simulink model "MPCmodel"  (R2023b)
settings: Solver=VariableStepAuto  StartTime=0.0  StopTime=10.0  RelTol=1e-3
libraries: aerolibanimutils x1
settings Model: Creator=Lingf  LastModifiedBy=deandre
settings SolverCC: AlgebraicLoopSolver=TrustRegion
settings DebuggingCC: UnconnectedInputMsg=warning  UnconnectedOutputMsg=warning  UnconnectedLineMsg=warning
settings ModelReferenceCC: EnableRefExpFcnMdlSchedulingChecks=on
settings RTWCC: DLArmComputeVersion=19.05

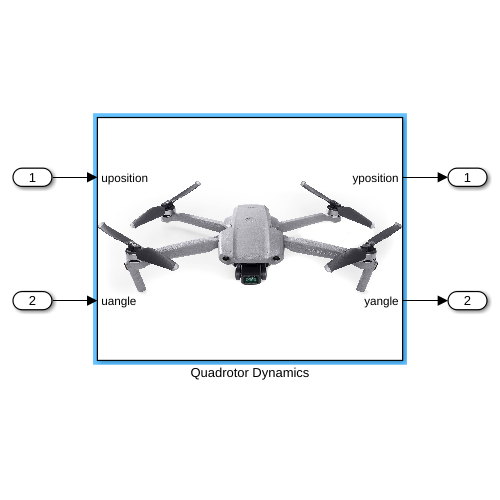
[thumbnail: Simulink's stored preview of the top-level diagram]
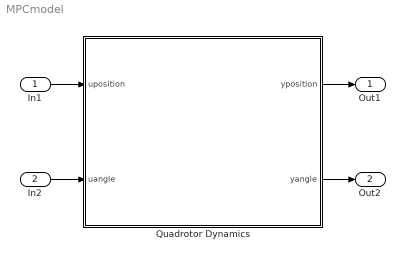
== system MPCmodel ==
  In1 : Inport
  In2 : Inport  Port=2
  Quadrotor Dynamics : Subsystem
      mask Display: image('$imagefile'); % Use "Edit Image" on toolstrip to change.
  Out1 : Outport
  Out2 : Outport  Port=2
  wires:
  In1/1 -> Quadrotor Dynamics/1(uposition)
  In2/1 -> Quadrotor Dynamics/2(uangle)
  Quadrotor Dynamics/1(yposition) -> Out1/1
  Quadrotor Dynamics/2(yangle) -> Out2/1

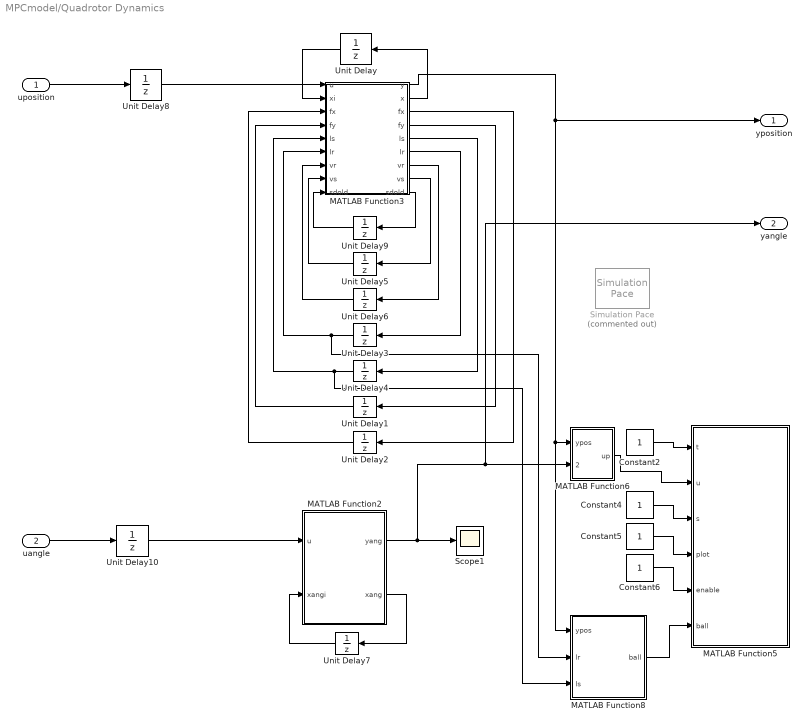
== system MPCmodel/Quadrotor Dynamics ==
  uposition : Inport
  uangle : Inport  Port=2
  Constant{2,4..6} (4 alike) : Constant
  MATLAB Function2 : MATLAB Function  TreatAsAtomicUnit=on
  MATLAB Function3 : MATLAB Function  TreatAsAtomicUnit=on
  MATLAB Function5 : MATLAB Function  TreatAsAtomicUnit=on
  MATLAB Function6 : MATLAB Function  TreatAsAtomicUnit=on
  MATLAB Function8 : MATLAB Function  TreatAsAtomicUnit=on
  Scope1 : Scope
  Simulation Pace : aerolibanimutils/Simulation Pace  Commented=on  SimulationPace=1  SleepMode=Auto  OutputPaceError=off  SampleTime=-1
  Unit Delay : UnitDelay  InitialCondition=|  SampleTime=-1  HasFrameUpgradeWarning=on
      | [0
      | 0
      | 0
      | 0
      | 1.50000000000000
      | 0]
  Unit Delay{1..6,9} (7 alike) : UnitDelay  SampleTime=-1  HasFrameUpgradeWarning=on
  Unit Delay10 : UnitDelay  InitialCondition=|  SampleTime=-1  HasFrameUpgradeWarning=on
      | [0
      | 0
      | 0]
  Unit Delay7 : UnitDelay  InitialCondition=|  SampleTime=-1  HasFrameUpgradeWarning=on
      | [0
      | 0
      | 0
      | 0
      | 0
      | 0]
  Unit Delay8 : UnitDelay  InitialCondition=|  SampleTime=-1  HasFrameUpgradeWarning=on
      | [0
      | 0
      | 0]
  yposition : Outport
  yangle : Outport  Port=2
  wires:
  Unit Delay6/1 -> MATLAB Function3/7("vr ")
  MATLAB Function3/2(x) -> Unit Delay/1
  MATLAB Function3/5(ls) -> Unit Delay4/1
  MATLAB Function2/1(yang) -> Scope1/1, yangle/1, MATLAB Function6/2(yang)
  Constant4/1 -> MATLAB Function5/3(s)
  Constant2/1 -> MATLAB Function5/1(t)
  MATLAB Function3/4(fy) -> Unit Delay1/1
  Unit Delay/1 -> MATLAB Function3/2(xi)
  MATLAB Function3/9(sdold) -> Unit Delay9/1
  MATLAB Function8/1(ball) -> MATLAB Function5/6(ball)
  Unit Delay4/1 -> MATLAB Function8/3(ls), MATLAB Function3/5("ls ")
  Unit Delay2/1 -> MATLAB Function3/3("fx ")
  MATLAB Function2/2(xang) -> Unit Delay7/1
  MATLAB Function3/1(y) -> yposition/1, MATLAB Function8/1(ypos), MATLAB Function6/1(ypos)
  MATLAB Function3/6(lr) -> Unit Delay3/1
  Constant5/1 -> MATLAB Function5/4(plot)
  MATLAB Function3/8(vs) -> Unit Delay5/1
  Unit Delay3/1 -> MATLAB Function8/2(lr), MATLAB Function3/6("lr ")
  Unit Delay5/1 -> MATLAB Function3/8("vs ")
  Constant6/1 -> MATLAB Function5/5(enable)
  MATLAB Function6/1(up) -> MATLAB Function5/2(u)
  Unit Delay7/1 -> MATLAB Function2/2(xangi)
  MATLAB Function3/7(vr) -> Unit Delay6/1
  MATLAB Function3/3(fx) -> Unit Delay2/1
  Unit Delay9/1 -> MATLAB Function3/9("sdold ")
  Unit Delay1/1 -> MATLAB Function3/4("fy ")
  uposition/1 -> Unit Delay8/1
  uangle/1 -> Unit Delay10/1
  Unit Delay8/1 -> MATLAB Function3/1(u)
  Unit Delay10/1 -> MATLAB Function2/1(u)

== matlab function MPCmodel/Quadrotor Dynamics/MATLAB Function2 ==
  data: yang output; xang output; u input; xangi input
function [yang,xang]= sysang(u,xangi)
Ts = 1/40;
g = 9.81;
A = [1,0.0250000000000000,0,0,0,0;0,1,0,0,0,0;0,0,1,0.0250000000000000,0,0;0,0,0,1,0,0;0,0,0,0,1,0.0250000000000000;0,0,0,0,0,1];
B = [0.0416666666666667,0,0;3.33333333333333,0,0;0,0.0416666666666667,0;0,3.33333333333333,0;0,0,0.0240384615384615;0,0,1.92307692307692];
C = [1,0,0,0,0,0;0,0,1,0,0,0;0,0,0,0,1,0];
D = zeros(3,3);
xang = zeros(6,1);
yang = zeros(3,1);
xang = A*xangi + B*u;
yang = C*xang + D*u;

== matlab function MPCmodel/Quadrotor Dynamics/MATLAB Function3 ==
  data: y output; x output; u input; xi input; fx input; fy input; fx output; fy output; ls input; lr input; ls output; lr output; vr input; vs input; vr output; vs output; sdold input; sdold output
function [y,x, fx,fy,ls,lr,vr,vs,sdold]= syspos(u,xi,fx,fy,ls,lr,vr,vs,sdold)
Ts = 1/40;
g = 9.81;
A = [1 0.025 0 0 0 0;0 1 0 0 0 0;0 0 1 0.025 0 0;0 0 0 1 0 0;0 0 0 0 1 0.025;0 0 0 0 0 1];
B = [-0.003065625 0 0;-0.24525 0 0;0 0.003065625 0;0 0.24525 0;0 0 0.0003125;0 0 0.025];
C = [1 0 0 0 0 0;0 0 1 0 0 0;0 0 0 0 1 0];
D = zeros(3,3);
x = zeros(6,1);
y = zeros(3,1);
x = A*xi + B*u;
y = C*x + D*u;
x(2) = x(2) - fx;
x(4) = x(4) - fy;


xdold = x(2)-xi(2);
ydold = x(4)-xi(4);
zdold = x(6)-xi(6);

yita = sqrt(0.5^2-lr^2-ls^2);
vrold = vr;
vsold = vs;
vr = ( yita^4*xdold - lr*yita^3*zdold + lr*ls*yita^2*sdold +...
    (lr*0.5^2-lr*ls^2)*vr^2 +...
    (lr*0.5^2-lr^3)*vs^2 +...
    2*vr*vs*lr^2*ls + lr*g*yita^3 )/((ls^2-0.5^2)*yita^2);
lr = lr + vr*Ts;
rdold = vr-vrold;

vs = ( yita^4*ydold - ls*yita^3*zdold + lr*ls*yita^2*rdold +...
    (ls*0.5^2-ls*lr^2)*vs^2 +...
    (ls*0.5^2-ls^3)*vr^2 +...
    2*vr*vs*ls^2*lr + ls*g*yita^3 )/((lr^2-0.5^2)*yita^2);
ls = ls + vs*Ts;
% sdold = vs(1,i+1);
sdold = vs(1)-vsold(1);

fx = 0.3*(xdold+rdold);
fy = 0.3*(ydold+sdold);

== matlab function MPCmodel/Quadrotor Dynamics/MATLAB Function5 ==
  data: t input; u input; s input; plot input; enable input; ball input
function qd_plot(t,u,s, plot, enable,ball)
    quad.nrotors =4;
    quad.d = 0.17;
    quad.r = 0.1;
    
    a1s = zeros(1, quad.nrotors);
    b1s = zeros(1, quad.nrotors);

    
    % vehicle dimensons
    d = quad.d; %Hub displacement from COG
    r = quad.r; %Rotor radius
    D = zeros(3,4);
    C = zeros(3,4);
    for i = 1:quad.nrotors
        theta = (i-1)/quad.nrotors*2*pi;
        %   Di      Rotor hub displacements (1x3)
        % first rotor is on the x-axis, clockwise order looking down from above
        D(:,i) = [ d*cos(theta); d*sin(theta); 0];
%         scal = s(1)/4;
        scal = 0.2/4;
        %Attitude center displacements
        C(:,i) = [ scal*cos(theta); scal*sin(theta); 0];
    end
    
    if enable == 1
        %draw ground
        figure(1);
        clf;
        if length(s) == 1
            axis([-0.5 1.5 -0.5 1.5 0 2]);
        else
%             axis([-s(1) s(1) -s(1) s(1) 0 s(2)])
            axis([-0.5 s(1) -0.5 s(1) 0 s(2)])
            s = 1.5;
        end
        hold on;
        
        % plot the ground boundaries and the big cross
        plot3([-0.5 -0.5],[-0.5 1],[0 0],'-b')
        plot3([-0.5 1.5],[-0.5 -0.5],[0 0],'-b')
        plot3([-0.5 1.5],[-0.5 1.5],[0 0],'-b')
        plot3([1.5 -0.5],[1.5 1.5],[0 0],'-b')
        plot3([1.5 1.5],[1.5 -0.5],[0 0],'-b')
        plot3([-0.5 1.5],[1.5 -0.5],[0 0],'-b')
        
        plot3([0 1], [0 0], [1.5 1.5],':r','LineWidth',0.2)
        plot3([1 1], [0 1], [1.5 1.5],':r','LineWidth',0.2)
        plot3([0 1], [1 1], [1.5 1.5],':r','LineWidth',0.2)
        plot3([0 0], [0 1], [1.5 1.5],':r','LineWidth',0.2)
        
        plot3([0 1], [0 0], [1 1],':r','LineWidth',0.2)
        plot3([1 1], [0 1], [1 1],':r','LineWidth',0.2)
        plot3([0 1], [1 1], [1 1],':r','LineWidth',0.2)
        plot3([0 0], [0 1], [1 1],':r','LineWidth',0.2)
        %READ STATE
        z = [u(1);u(2);u(3)];
        n = [u(4);u(5);u(6)];
        
        %PREPROCESS ROTATION MATRIX
        phi = n(1);    %Euler angles
        the = n(2);
        psi = n(3);
        
        R = [cos(the)*cos(phi) sin(psi)*sin(the)*cos(phi)-cos(psi)*sin(phi) cos(psi)*sin(the)*cos(phi)+sin(psi)*sin(phi);   %BBF > Inertial rotation matrix
            cos(the)*sin(phi) sin(psi)*sin(the)*sin(phi)+cos(psi)*cos(phi) cos(psi)*sin(the)*sin(phi)-sin(psi)*cos(phi);
            -sin(the)         sin(psi)*cos(the)                            cos(psi)*cos(the)];
        
        %Manual Construction
        %Q3 = [cos(psi) -sin(psi) 0;sin(psi) cos(psi) 0;0 0 1];   %Rotation mappings
        %Q2 = [cos(the) 0 sin(the);0 1 0;-sin(the) 0 cos(the)];
        %Q1 = [1 0 0;0 cos(phi) -sin(phi);0 sin(phi) cos(phi)];
        %R = Q3*Q2*Q1;    %Rotation matrix
        
        %CALCULATE FLYER TIP POSITONS USING COORDINATE FRAME ROTATION
        F = [1 0 0;0 -1 0;0 0 -1];
        
        %Draw flyer rotors
        t = [0:pi/8:2*pi];
        circle = zeros(3,17);
        for j = 1:length(t)
            circle(:,j) = [r*sin(t(j));r*cos(t(j));0];
        end
        hub = zeros(3,4);
        tippath = zeros(3,17,4);
        for i = 1:quad.nrotors
            hub(:,i) = F*(z + R*D(:,i)); %points in the inertial frame
            center = F*z;
            ball_pos = F*ball;
            plot3(center(1),center(2),center(3),'r.')
            plot3(ball_pos(1),ball_pos(2),ball_pos(3),'co')
            plot3([center(1) ball_pos(1)],[center(2) ball_pos(2)],[center(3) ball_pos(3)],'-b')
            
            q = 1; %Flapping angle scaling for output display - makes it easier to see what flapping is occurring
            Rr = [cos(q*a1s(i))  sin(q*b1s(i))*sin(q*a1s(i)) cos(q*b1s(i))*sin(q*a1s(i));   %Rotor > Plot frame
                0              cos(q*b1s(i))               -sin(q*b1s(i));
                -sin(q*a1s(i)) sin(q*b1s(i))*cos(q*a1s(i)) cos(q*b1s(i))*cos(q*a1s(i))];
            
            tippath(:,:,i) = F*R*Rr*circle;
            plot3([hub(1,i)+tippath(1,:,i)],[hub(2,i)+tippath(2,:,i)],[hub(3,i)+tippath(3,:,i)],'b-')
        end
        
        %Draw flyer
        hub0 = F*z;  % centre of vehicle
        for i = 1:quad.nrotors
            % line from hub to centre plot3([hub(1,N) hub(1,S)],[hub(2,N) hub(2,S)],[hub(3,N) hub(3,S)],'-b')
            plot3([hub(1,i) hub0(1)],[hub(2,i) hub0(2)],[hub(3,i) hub0(3)],'-b')
            
            % plot a circle at the hub itself
            plot3([hub(1,i)],[hub(2,i)],[hub(3,i)],'o')
        end
        
        % plot the vehicle's centroid on the ground plane
        plot3([z(1) 0],[-z(2) 0],[0 0],'--k')
        plot3([z(1)],[-z(2)],[0],'xk')
        plot3([z(1) z(1)],[-z(2) -s],[0 0],'r-.')

        % label the axes
        xlabel('x');
        ylabel('y');
        zlabel('z (height above ground)');
        view([-5 -2 5]);
    end;

== matlab function MPCmodel/Quadrotor Dynamics/MATLAB Function6 ==
  data: up output; ypos input; yang input
function up= upp(ypos,yang)
up = [ypos(1) -ypos(2) -ypos(3) yang(1) yang(2) yang(3)];

== matlab function MPCmodel/Quadrotor Dynamics/MATLAB Function8 ==
  data: ball output; ypos input; lr input; ls input
function ball= balll(ypos,lr,ls)
ball=[ypos(1)+lr(1) -(ypos(2)+ls(1)) 1-ypos(3)-sqrt(0.25-lr(1)^2-ls(1)^2)]';
